simulink model "ec_datadict_buses"  (Simulink 10.0)
settings: Solver=FixedStepDiscrete  StartTime=0.0  StopTime=10  RelTol=1e-3  EnableMultiTasking=on
PreLoadFcn:
  | ec_data_fixpt_sc;
StartFcn:
  | tic
StopFcn:
  | toc
undefined symbols (not defined in the file): dfilt, ec_length, ec_window_len, Fs, magnitude, pic_frame_size, spkr_to_mic_filter, spkr_to_mic_gain
libraries: dspsrcs4 x24, simulink x14, dsparch4 x4, dspobslib x3, dspsnks4 x3, dspbuff3 x3, dspwin32 x2, dspsigops x2, dspmathops x2, dspadpt3 x1
settings Model: Creator=Kerry Schutz  LastModifiedBy=bhisma
settings DataIOCC: LimitDataPoints=on  SaveFormat=Structure  SignalLoggingSaveFormat=ModelDataLogs  SignalLogging=off
settings OptimizationCC: BlockReduction=off  DefaultParameterBehavior=Inlined  ExpressionDepthLimit=2147483647  InitFltsAndDblsToZero=on  LifeSpan=1  EfficientTunableParamExpr=on
settings DebuggingCC: SaveWithParameterizedLinksMsg=none  SolverPrmCheckMsg=warning  FcnCallInpInsideContextMsg=warning  StateNameClashWarn=warning
settings HardwareCC: ProdBitPerInt=16  ProdWordSize=16  ProdHWDeviceType=Specified
settings SFSimCC: SimUseLocalCustomCode=on  MATLABDynamicMemAlloc=off  CustomCodeUndefinedFunction=FilterOut
settings RTWCC: Description=Real-Time Workshop Embedded Coder (no auto configuration)  SystemTargetFile=ert.tlc  GenCodeOnly=on  TemplateMakefile=ert_default_tmf  GenerateReport=on  RTWUseLocalCustomCode=on  IncludeHyperlinkInReport=on  LaunchReport=on
settings CodeAppCC: IgnoreCustomStorageClasses=off  CustomSymbolStrType=$N$R$M  InternalIdentifier=Classic
settings ERTTargetCC: TargetFcnLib=ansi_tfl_tmw.mat  GenerateSampleERTMain=on  IncludeMdlTerminateFcn=off  SupportAbsoluteTime=off  SupportNonFinite=off  SupportComplex=off  InlinedParameterPlacement=NonHierarchical  ERTCustomFileTemplate=example_file_process.tlc  ConvertIfToSwitch=off  SuppressUnreachableDefaultCases=off

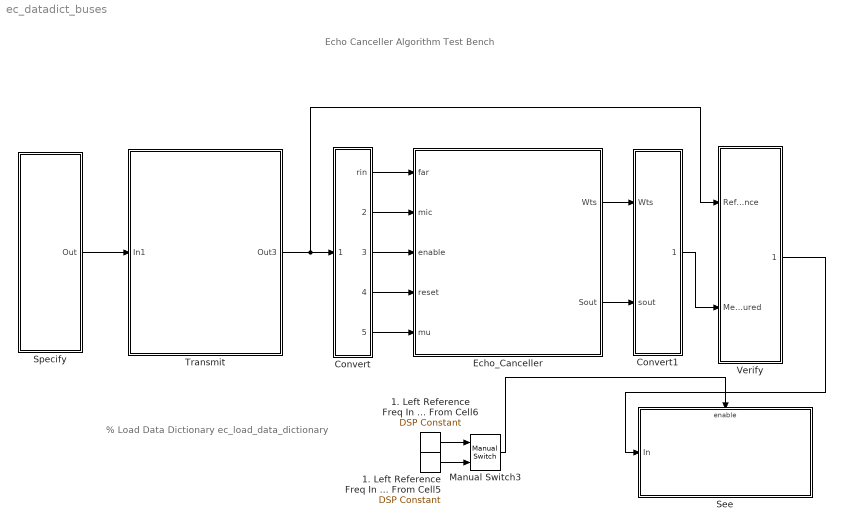
== system ec_datadict_buses ==
  note: Echo Canceller
      | Algorithm Test Bench
  note: % Load Data Dictionary
      | ec_load_data_dictionary
  1. Left Reference Freq In Hz From Cell5 : dspsrcs4/DSP Constant  SystemSampleTime=-1  Value=0  SampleMode=Discrete  discreteOutput=Sample-based  continuousOutput=Sample-based  sampTime=pic_frame_size/Fs  framePeriod=pic_frame_size/Fs  dataType=double  isSigned=on  wordLen=16  udDataType=sfix(16)  fracBitsMode=Best precision  numFracBits=15  InterpretAs1D=-inf  Ts=-inf  FramebasedOutput=-inf
      settings: SourceProductName=DSP System Toolbox  SourceProductBaseCode=DS  additionalParams=on
  1. Left Reference Freq In Hz From Cell6 : dspsrcs4/DSP Constant  SystemSampleTime=-1  Value=1  SampleMode=Discrete  discreteOutput=Sample-based  continuousOutput=Sample-based  sampTime=pic_frame_size/Fs  framePeriod=pic_frame_size/Fs  dataType=double  isSigned=on  wordLen=16  udDataType=sfix(16)  fracBitsMode=Best precision  numFracBits=15  InterpretAs1D=-inf  Ts=-inf  FramebasedOutput=-inf
      settings: SourceProductName=DSP System Toolbox  SourceProductBaseCode=DS  additionalParams=on
  Convert : Subsystem
  Convert1 : Subsystem
  Echo_Canceller : Subsystem  MinMaxOverflowLogging=MinMaxAndOverflow
      mask Display: image(imread('dsp_art.bmp'))
  Manual Switch3 : simulink/Signal Routing/Manual Switch  SystemSampleTime=-1  sw=1  action=0  varsize=off
      settings: SourceProductName=Simulink  SourceProductBaseCode=SL
  See : Subsystem
      mask Display: image(imread('visualizations.bmp'))
  Specify : Subsystem
      mask Display: image(imread('tests.bmp'))
  Transmit : Subsystem
      mask Display: image(imread('trans_path.bmp'))
  Verify : Subsystem
      mask Display: image(imread('verifications.bmp'))
  wires:
  Specify/1(Out) -> Transmit/1(In1)
  Transmit/1(Out3) -> Convert/1("  "), Verify/1(Reference)
  Convert/1(rin) -> Echo_Canceller/1(" far ")
  Convert/2(sin) -> Echo_Canceller/2("  mic")
  Convert/3(enable) -> Echo_Canceller/3(" enable")
  Echo_Canceller/1(Wts) -> Convert1/1(Wts)
  Echo_Canceller/2(Sout) -> Convert1/2(sout)
  Convert1/1(" ") -> Verify/2(Measured)
  Verify/1("  ") -> See/1(In)
  Convert/5(mu) -> Echo_Canceller/5(mu)
  Convert/4(reset) -> Echo_Canceller/4(reset)
  Manual Switch3/1 -> See/Enable
  1. Left Reference Freq In Hz From Cell5/1 -> Manual Switch3/2
  1. Left Reference Freq In Hz From Cell6/1 -> Manual Switch3/1

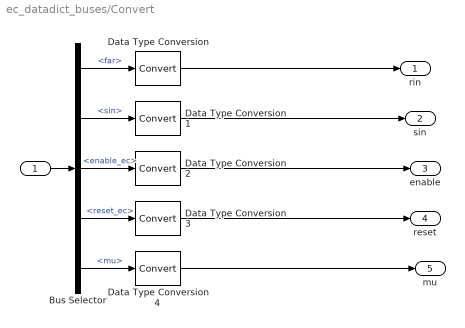
== system ec_datadict_buses/Convert ==
  "  " : Inport
  Bus Selector : BusSelector  OutputSignals=far,sin,enable_ec,reset_ec,mu
  Data Type Conversion{,1..4} (5 alike) : DataTypeConversion  SaturateOnIntegerOverflow=on
  rin : Outport
  sin : Outport  Port=2
  enable : Outport  Port=3
  reset : Outport  Port=4
  mu : Outport  Port=5
  wires:
  Bus Selector/1 -> Data Type Conversion/1  "<far>"
  Bus Selector/2 -> Data Type Conversion1/1  "<sin>"
  "  "/1 -> Bus Selector/1
  Data Type Conversion1/1 -> sin/1
  Data Type Conversion/1 -> rin/1
  Bus Selector/3 -> Data Type Conversion2/1  "<enable_ec>"
  Data Type Conversion2/1 -> enable/1
  Bus Selector/4 -> Data Type Conversion3/1  "<reset_ec>"
  Data Type Conversion3/1 -> reset/1
  Bus Selector/5 -> Data Type Conversion4/1  "<mu>"
  Data Type Conversion4/1 -> mu/1

== system ec_datadict_buses/Convert1 ==
  Wts : Inport
  sout : Inport  Port=2
  Bus Creator : BusCreator  Inputs=2
  Data Type Conversion : DataTypeConversion  OutDataTypeStr=double  SaturateOnIntegerOverflow=on
  Data Type Conversion1 : DataTypeConversion  OutDataTypeStr=double  SaturateOnIntegerOverflow=on
  " " : Outport
  wires:
  Wts/1 -> Data Type Conversion/1
  Bus Creator/1 -> " "/1
  sout/1 -> Data Type Conversion1/1
  Data Type Conversion/1 -> Bus Creator/1  "Wts"
  Data Type Conversion1/1 -> Bus Creator/2  "sout"

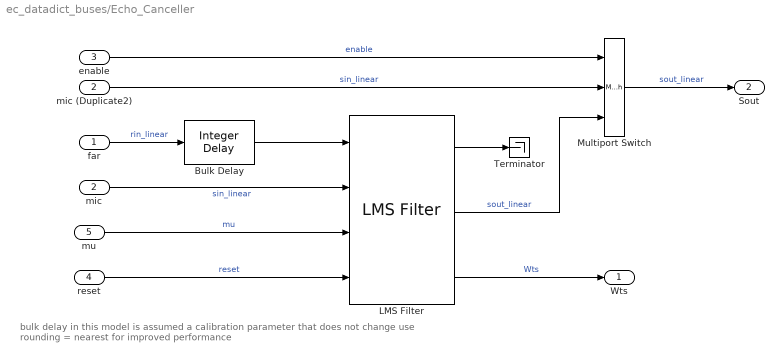
== system ec_datadict_buses/Echo_Canceller ==
  note: bulk delay in this model is assumed a calibration parameter that does not change
      | use rounding = nearest for improved performance
  " far " : Inport
  "  mic" : Inport  Port=2
  " enable" : Inport  Port=3
  reset : Inport  Port=4
  mu : Inport  Port=5
  "  mic (Duplicate2)" : InportShadow  Port=2
  Bulk Delay : dspobslib/Integer Delay  delay=spkr_to_mic_delay % this compensates for the delay in the filter and the spkr to mic path  ic=0  reset_popup=None
      settings: SourceProductName=DSP System Toolbox  SourceProductBaseCode=DS
  LMS Filter : dspadpt3/LMS Filter  Algo=LMS  L=ec_length  stepflag=Input port  mu=0.1  leakage=1.0  ic=0  Adapt=off  resetflag=Non-zero sample  weights=on  addnparflag=off  roundingMode=Nearest  overflowMode=off  secondCoeffMode=Binary point scaling  secondCoeffWordLength=2  secondCoeffFracLength=15  memoryMode=Binary point scaling  memoryWordLength=LMS_Wts_WordLen  memoryFracLength=LMS_Wts_FracLen  prodOutputMode=Binary point scaling  prodOutputWordLength=LMS_Prod_WordLen  prodOutputFracLength=20  prodOutput2Mode=Binary point scaling  prodOutput2FracLength=LMS_Prod_FracLen  prodOutput3Mode=Binary point scaling  prodOutput3FracLength=LMS_Prod_FracLen  prodOutput4Mode=Binary point scaling  prodOutput4FracLength=LMS_Prod_FracLen  quotientMode=Binary point scaling  quotientFracLength=20  accumMode=Binary point scaling  accumWordLength=LMS_Accum_WordLen  accumFracLength=20  accum2Mode=Binary point scaling  accum2FracLength=LMS_Accum_FracLen
      settings: SourceProductName=DSP System Toolbox  SourceProductBaseCode=DS
  Multiport Switch : MultiPortSwitch  DataPortOrder=Zero-based contiguous  Inputs=2  zeroidx=on
  Terminator : Terminator
  Wts : Outport
  Sout : Outport  Port=2
  wires:
  " far "/1 -> Bulk Delay/1  "rin_linear"
  "  mic"/1 -> LMS Filter/2  "sin_linear"
  LMS Filter/3 -> Wts/1  "Wts"
  LMS Filter/1 -> Terminator/1
  " enable"/1 -> Multiport Switch/1  "enable"
  LMS Filter/2 -> Multiport Switch/3  "sout_linear"
  "  mic (Duplicate2)"/1 -> Multiport Switch/2  "sin_linear"
  reset/1 -> LMS Filter/4  "reset"
  Multiport Switch/1 -> Sout/1  "sout_linear"
  mu/1 -> LMS Filter/3  "mu"
  Bulk Delay/1 -> LMS Filter/1

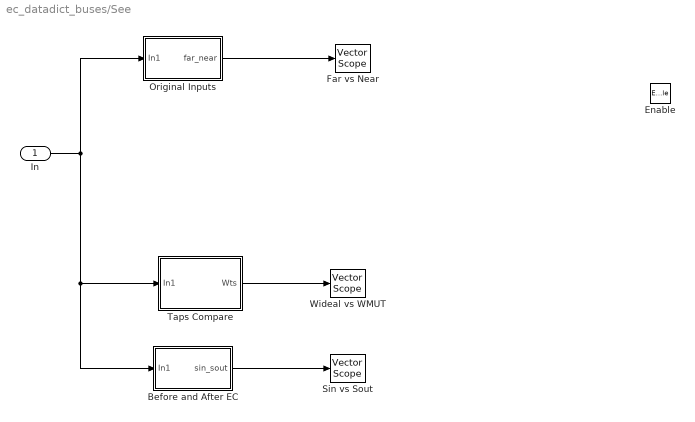
== system ec_datadict_buses/See ==
  In : Inport
  Enable : EnablePort
  Before and After EC : Subsystem
  Far vs Near : dspsnks4/Vector Scope  ScopeProperties=on  Domain=Time  HorizSpan=1  DisplayProperties=off  AxisGrid=on  Memory=off  FrameNumber=on  AxisLegend=off  AxisZoom=off  OpenScopeAtSimStart=on  OpenScopeImmediately=off  FigPos=[41 300 287 179]  AxisProperties=off  XUnits=Hertz  XRange=[0...Fs/2]  InheritXIncr=on  XIncr=1  XLabel=Time  XLimit=Auto  XMin=0  XMax=1  XStart=0  YUnits=dB  YLabel=Amplitude  LineProperties=off  LineColors=r|g
      settings: SourceProductName=DSP System Toolbox  SourceProductBaseCode=DS  YMin=-0.904474745892036  YMax=0.903014948842516
  Original Inputs : Subsystem
  Sin vs Sout : dspsnks4/Vector Scope  ScopeProperties=on  Domain=Time  HorizSpan=1  DisplayProperties=off  AxisGrid=on  Memory=off  FrameNumber=on  AxisLegend=off  AxisZoom=off  OpenScopeAtSimStart=on  OpenScopeImmediately=off  FigPos=[339 300 287 179]  AxisProperties=off  XUnits=Hertz  XRange=[0...Fs/2]  InheritXIncr=on  XIncr=1  XLabel=Time  XLimit=Auto  XMin=0  XMax=1  XStart=0  YUnits=dB  YLabel=Amplitude  LineProperties=off  LineColors=r|g
      settings: SourceProductName=DSP System Toolbox  SourceProductBaseCode=DS  YMin=-0.904474745892036  YMax=0.903014948842516
  Taps Compare : Subsystem
  Wideal vs WMUT : dspsnks4/Vector Scope  ScopeProperties=on  Domain=Time  HorizSpan=1  DisplayProperties=off  AxisGrid=on  Memory=off  FrameNumber=on  AxisLegend=off  AxisZoom=off  OpenScopeAtSimStart=on  OpenScopeImmediately=off  FigPos=[637 300 318 179]  AxisProperties=off  XUnits=Hertz  XRange=[0...Fs/2]  InheritXIncr=on  XIncr=1  XLabel=Time  XLimit=User-defined  XMin=4  XMax=6  XStart=0  YUnits=dB  YLabel=Amplitude  LineProperties=off  LineColors=r|g
      settings: SourceProductName=DSP System Toolbox  SourceProductBaseCode=DS  YMin=-0.0718456241378401  YMax=0.392086848285075
  wires:
  Original Inputs/1(far_near) -> Far vs Near/1
  In/1 -> Original Inputs/1(In1), Taps Compare/1(In1), Before and After EC/1(In1)
  Taps Compare/1(Wts) -> Wideal vs WMUT/1
  Before and After EC/1(sin_sout) -> Sin vs Sout/1

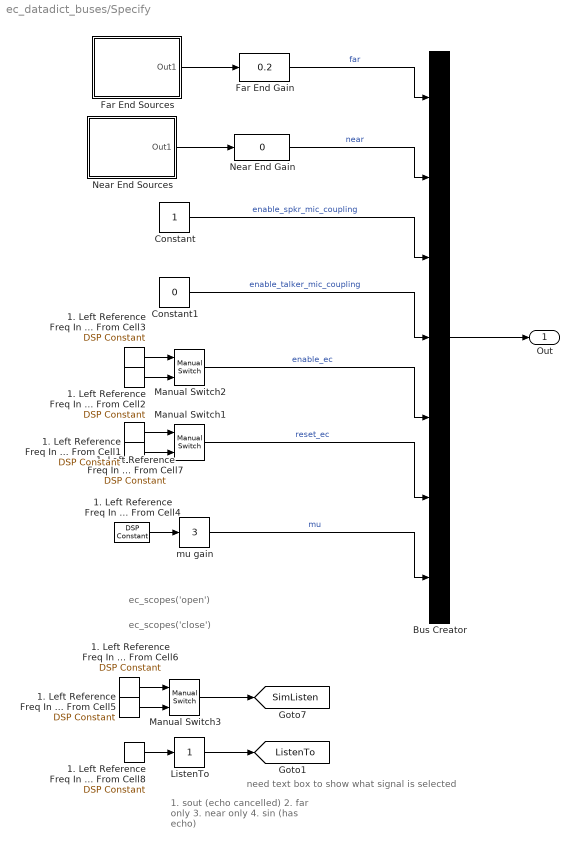
== system ec_datadict_buses/Specify ==
  note: ec_scopes('open')
  note: ec_scopes('close')
  note: need text box to show what signal is selected
  note: 1. sout (echo cancelled)
      | 2. far only
      | 3. near only
      | 4. sin (has echo)
  1. Left Reference Freq In Hz From Cell1 : dspsrcs4/DSP Constant  SystemSampleTime=-1  Value=0  SampleMode=Discrete  discreteOutput=Sample-based  continuousOutput=Sample-based  sampTime=pic_frame_size/Fs  framePeriod=pic_frame_size/Fs  dataType=double  isSigned=on  wordLen=16  udDataType=sfix(16)  fracBitsMode=Best precision  numFracBits=15  InterpretAs1D=-inf  Ts=-inf  FramebasedOutput=-inf
      settings: SourceProductName=DSP System Toolbox  SourceProductBaseCode=DS  additionalParams=on
  1. Left Reference Freq In Hz From Cell2 : dspsrcs4/DSP Constant  SystemSampleTime=-1  Value=0  SampleMode=Discrete  discreteOutput=Sample-based  continuousOutput=Sample-based  sampTime=pic_frame_size/Fs  framePeriod=pic_frame_size/Fs  dataType=double  isSigned=on  wordLen=16  udDataType=sfix(16)  fracBitsMode=Best precision  numFracBits=15  InterpretAs1D=-inf  Ts=-inf  FramebasedOutput=-inf
      settings: SourceProductName=DSP System Toolbox  SourceProductBaseCode=DS  additionalParams=on
  1. Left Reference Freq In Hz From Cell3 : dspsrcs4/DSP Constant  SystemSampleTime=-1  Value=1  SampleMode=Discrete  discreteOutput=Sample-based  continuousOutput=Sample-based  sampTime=pic_frame_size/Fs  framePeriod=pic_frame_size/Fs  dataType=double  isSigned=on  wordLen=16  udDataType=sfix(16)  fracBitsMode=Best precision  numFracBits=15  InterpretAs1D=-inf  Ts=-inf  FramebasedOutput=-inf
      settings: SourceProductName=DSP System Toolbox  SourceProductBaseCode=DS  additionalParams=on
  1. Left Reference Freq In Hz From Cell4 : dspsrcs4/DSP Constant  SystemSampleTime=-1  Value=.001  SampleMode=Discrete  discreteOutput=Sample-based  continuousOutput=Sample-based  sampTime=pic_frame_size/Fs  framePeriod=2  dataType=double  isSigned=on  wordLen=16  udDataType=sfix(16)  fracBitsMode=Best precision  numFracBits=15  InterpretAs1D=-inf  Ts=-inf  FramebasedOutput=-inf
      settings: SourceProductName=DSP System Toolbox  SourceProductBaseCode=DS  additionalParams=on
  1. Left Reference Freq In Hz From Cell5 : dspsrcs4/DSP Constant  SystemSampleTime=-1  Value=0  SampleMode=Discrete  discreteOutput=Sample-based  continuousOutput=Sample-based  sampTime=pic_frame_size/Fs  framePeriod=pic_frame_size/Fs  dataType=double  isSigned=on  wordLen=16  udDataType=sfix(16)  fracBitsMode=Best precision  numFracBits=15  InterpretAs1D=-inf  Ts=-inf  FramebasedOutput=-inf
      settings: SourceProductName=DSP System Toolbox  SourceProductBaseCode=DS  additionalParams=on
  1. Left Reference Freq In Hz From Cell6 : dspsrcs4/DSP Constant  SystemSampleTime=-1  Value=1  SampleMode=Discrete  discreteOutput=Sample-based  continuousOutput=Sample-based  sampTime=pic_frame_size/Fs  framePeriod=pic_frame_size/Fs  dataType=double  isSigned=on  wordLen=16  udDataType=sfix(16)  fracBitsMode=Best precision  numFracBits=15  InterpretAs1D=-inf  Ts=-inf  FramebasedOutput=-inf
      settings: SourceProductName=DSP System Toolbox  SourceProductBaseCode=DS  additionalParams=on
  1. Left Reference Freq In Hz From Cell7 : dspsrcs4/DSP Constant  SystemSampleTime=-1  Value=1  SampleMode=Discrete  discreteOutput=Sample-based  continuousOutput=Sample-based  sampTime=pic_frame_size/Fs  framePeriod=pic_frame_size/Fs  dataType=double  isSigned=on  wordLen=16  udDataType=sfix(16)  fracBitsMode=Best precision  numFracBits=15  InterpretAs1D=-inf  Ts=-inf  FramebasedOutput=-inf
      settings: SourceProductName=DSP System Toolbox  SourceProductBaseCode=DS  additionalParams=on
  1. Left Reference Freq In Hz From Cell8 : dspsrcs4/DSP Constant  SystemSampleTime=-1  Value=1  SampleMode=Discrete  discreteOutput=Sample-based  continuousOutput=Sample-based  sampTime=pic_frame_size/Fs  framePeriod=2  dataType=double  isSigned=on  wordLen=16  udDataType=sfix(16)  fracBitsMode=Best precision  numFracBits=15  InterpretAs1D=-inf  Ts=-inf  FramebasedOutput=-inf
      settings: SourceProductName=DSP System Toolbox  SourceProductBaseCode=DS  additionalParams=on
  Bus Creator : BusCreator  Inputs=7
  Constant : Constant
  Constant1 : Constant  Value=0
  Far End Gain : simulink/Math Operations/Slider Gain  SystemSampleTime=-1  low=0  gain=0.2  high=10
  Far End Sources : Subsystem
  ListenTo : simulink/Math Operations/Slider Gain  SystemSampleTime=-1  low=0  gain=1  high=10
  Manual Switch1 : simulink/Signal Routing/Manual Switch  SystemSampleTime=-1  sw=0  action=0  varsize=off
      settings: SourceProductName=Simulink  SourceProductBaseCode=SL
  Manual Switch2 : simulink/Signal Routing/Manual Switch  SystemSampleTime=-1  sw=1  action=0  varsize=off
      settings: SourceProductName=Simulink  SourceProductBaseCode=SL
  Manual Switch3 : simulink/Signal Routing/Manual Switch  SystemSampleTime=-1  sw=0  action=0  varsize=off
      settings: SourceProductName=Simulink  SourceProductBaseCode=SL
  Near End Gain : simulink/Math Operations/Slider Gain  SystemSampleTime=-1  low=0  gain=0  high=10
  Near End Sources : Subsystem
  mu gain : simulink/Math Operations/Slider Gain  SystemSampleTime=-1  low=0  gain=3  high=100
  Out : Outport
  tag scope: ListenTo=global, SimListen=global
  wires:
  Far End Sources/1(Out1) -> Far End Gain/1
  Near End Sources/1(Out1) -> Near End Gain/1
  Far End Gain/1 -> Bus Creator/1  "far"
  Near End Gain/1 -> Bus Creator/2  "near"
  Bus Creator/1 -> Out/1
  Constant/1 -> Bus Creator/3  "enable_spkr_mic_coupling"
  Constant1/1 -> Bus Creator/4  "enable_talker_mic_coupling"
  1. Left Reference Freq In Hz From Cell1/1 -> Manual Switch1/2
  1. Left Reference Freq In Hz From Cell7/1 -> Manual Switch1/1
  Manual Switch1/1 -> Bus Creator/6  "reset_ec"
  1. Left Reference Freq In Hz From Cell2/1 -> Manual Switch2/2
  1. Left Reference Freq In Hz From Cell3/1 -> Manual Switch2/1
  Manual Switch2/1 -> Bus Creator/5  "enable_ec"
  1. Left Reference Freq In Hz From Cell4/1 -> mu gain/1
  mu gain/1 -> Bus Creator/7  "mu"
  1. Left Reference Freq In Hz From Cell5/1 -> Manual Switch3/2
  1. Left Reference Freq In Hz From Cell6/1 -> Manual Switch3/1
  Manual Switch3/1 -> [SimListen]
  ListenTo/1 -> [ListenTo]
  1. Left Reference Freq In Hz From Cell8/1 -> ListenTo/1

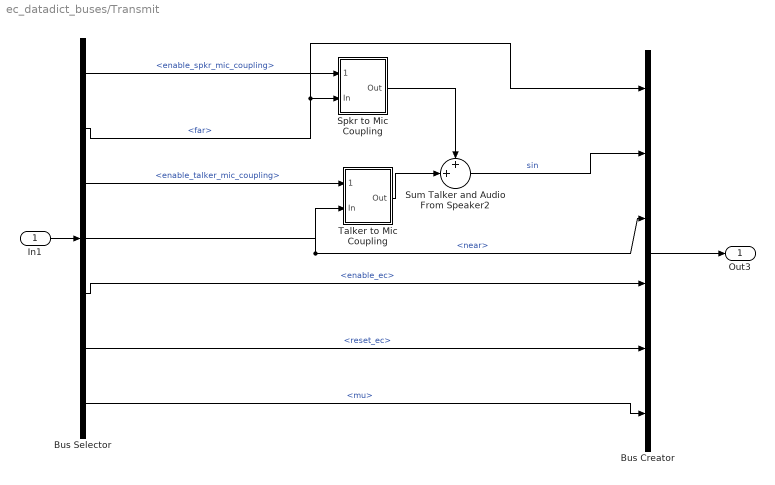
== system ec_datadict_buses/Transmit ==
  In1 : Inport
  Bus Creator : BusCreator  Inputs=6
  Bus Selector : BusSelector  OutputSignals=enable_spkr_mic_coupling,far,enable_talker_mic_coupling,near,enable_ec,reset_ec,mu
  Spkr to Mic Coupling : Subsystem
  Sum Talker and Audio From Speaker2 : Sum  Inputs=++|  SaturateOnIntegerOverflow=on  OutDataTypeStr=Inherit: Same as first input
  Talker to Mic Coupling : Subsystem
  Out3 : Outport
  wires:
  In1/1 -> Bus Selector/1
  Bus Creator/1 -> Out3/1
  Bus Selector/2 -> Spkr to Mic Coupling/2(In), Bus Creator/1  "<far>"
  Bus Selector/1 -> Spkr to Mic Coupling/1(enable)  "<enable_spkr_mic_coupling>"
  Bus Selector/3 -> Talker to Mic Coupling/1(enable)  "<enable_talker_mic_coupling>"
  Bus Selector/4 -> Talker to Mic Coupling/2(In), Bus Creator/3  "<near>"
  Spkr to Mic Coupling/1(Out) -> Sum Talker and Audio From Speaker2/1
  Talker to Mic Coupling/1(Out) -> Sum Talker and Audio From Speaker2/2
  Bus Selector/5 -> Bus Creator/4  "<enable_ec>"
  Bus Selector/6 -> Bus Creator/5  "<reset_ec>"
  Bus Selector/7 -> Bus Creator/6  "<mu>"
  Sum Talker and Audio From Speaker2/1 -> Bus Creator/2  "sin"

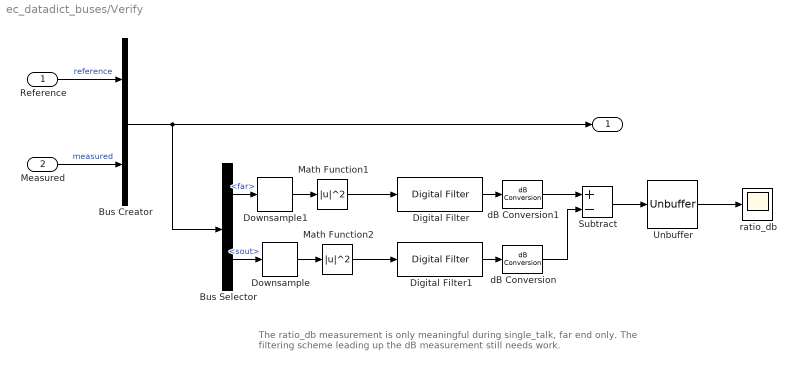
== system ec_datadict_buses/Verify ==
  note: The ratio_db measurement is only meaningful during single_talk, far end only.
      | The filtering scheme leading up the dB measurement still needs work.
  Reference : Inport
  Measured : Inport  Port=2
  Bus Creator : BusCreator  Inputs=2
  Bus Selector : BusSelector  OutputSignals=reference.far,measured.sout
  Digital Filter : dsparch4/Digital Filter  TypePopup=FIR (all zeros)  IIRFiltStruct=Direct form II transposed  AllPoleFiltStruct=Direct form  FIRFiltStruct=Direct form  CoeffSource=Specify via dialog  NumCoeffs=[ones(1,80)/80]  DenCoeffs=[1 0.1]  BiQuadCoeffs=[1 0.3 0.4 1 0.1 0.2]  LatticeCoeffs=[0.2 0.4]  denIgnore=on  FiltPerSampPopup=One filter per frame  IC=0  ICnum=0  ICden=0  roundingMode=Floor  overflowMode=off  ScaleValues=1  scaleValueFracLength=14  stageInFracLength=15  stageOutFracLength=15  FilterSource=Specify via dialog  dfiltObjectName=dfilt.dffir([1 2 1])
      settings: SourceProductName=DSP System Toolbox  SourceProductBaseCode=DS
  Digital Filter1 : dsparch4/Digital Filter  TypePopup=FIR (all zeros)  IIRFiltStruct=Direct form II transposed  AllPoleFiltStruct=Direct form  FIRFiltStruct=Direct form  CoeffSource=Specify via dialog  NumCoeffs=[ones(1,80)/80]  DenCoeffs=[1 0.1]  BiQuadCoeffs=[1 0.3 0.4 1 0.1 0.2]  LatticeCoeffs=[0.2 0.4]  denIgnore=on  FiltPerSampPopup=One filter per frame  IC=0  ICnum=0  ICden=0  roundingMode=Floor  overflowMode=off  ScaleValues=1  scaleValueFracLength=14  stageInFracLength=15  stageOutFracLength=15  FilterSource=Specify via dialog  dfiltObjectName=dfilt.dffir([1 2 1])
      settings: SourceProductName=DSP System Toolbox  SourceProductBaseCode=DS
  Downsample : dspsigops/Downsample  N=10  phase=0  ic=0  smode=Allow multirate  fmode=Maintain input frame size
      settings: SourceProductName=DSP System Toolbox  SourceProductBaseCode=DS
  Downsample1 : dspsigops/Downsample  N=10  phase=0  ic=0  smode=Allow multirate  fmode=Maintain input frame size
      settings: SourceProductName=DSP System Toolbox  SourceProductBaseCode=DS
  Math Function1 : Math  Operator=magnitude^2  SaturateOnIntegerOverflow=on
  Math Function2 : Math  Operator=magnitude^2  SaturateOnIntegerOverflow=on
  Subtract : Sum  Inputs=+-
  Unbuffer : dspbuff3/Unbuffer  ic=0
      settings: SourceProductName=DSP System Toolbox  SourceProductBaseCode=DS
  dB Conversion : dspmathops/dB Conversion  SystemSampleTime=-1  dBtype=dB  intype=Power  R=1  fuzz=on
      settings: SourceProductName=DSP System Toolbox
  dB Conversion1 : dspmathops/dB Conversion  SystemSampleTime=-1  dBtype=dB  intype=Power  R=1  fuzz=on
      settings: SourceProductName=DSP System Toolbox
  ratio_db : Scope
  "  " : Outport
  wires:
  Reference/1 -> Bus Creator/1  "reference"
  Measured/1 -> Bus Creator/2  "measured"
  Bus Creator/1 -> "  "/1, Bus Selector/1
  Bus Selector/1 -> Downsample1/1  "<far>"
  Bus Selector/2 -> Downsample/1  "<sout>"
  Unbuffer/1 -> ratio_db/1
  Math Function1/1 -> Digital Filter/1
  Digital Filter/1 -> dB Conversion1/1
  Math Function2/1 -> Digital Filter1/1
  Digital Filter1/1 -> dB Conversion/1
  Subtract/1 -> Unbuffer/1
  Downsample/1 -> Math Function2/1
  Downsample1/1 -> Math Function1/1
  dB Conversion/1 -> Subtract/2
  dB Conversion1/1 -> Subtract/1

== system ec_datadict_buses/See/Before and After EC ==
  In1 : Inport
  Bus Selector : BusSelector  OutputSignals=reference.sin,measured.sout
  Matrix Concatenate1 : Concatenate  Mode=Multidimensional array  ConcatenateDimension=2
  sin_sout : Outport
  wires:
  Matrix Concatenate1/1 -> sin_sout/1
  In1/1 -> Bus Selector/1
  Bus Selector/2 -> Matrix Concatenate1/2  "<sout>"
  Bus Selector/1 -> Matrix Concatenate1/1  "<sin>"

== system ec_datadict_buses/See/Original Inputs ==
  In1 : Inport
  Bus Selector : BusSelector  OutputSignals=reference.far,reference.near
  Matrix Concatenate1 : Concatenate  Mode=Multidimensional array  ConcatenateDimension=2
  far_near : Outport
  wires:
  Bus Selector/1 -> Matrix Concatenate1/1  "<far>"
  Bus Selector/2 -> Matrix Concatenate1/2  "<near>"
  In1/1 -> Bus Selector/1
  Matrix Concatenate1/1 -> far_near/1

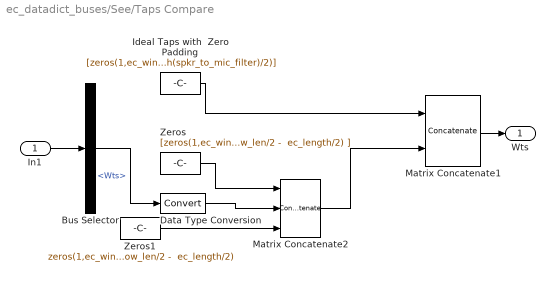
== system ec_datadict_buses/See/Taps Compare ==
  In1 : Inport
  Bus Selector : BusSelector  OutputSignals=measured.Wts
  Data Type Conversion : DataTypeConversion
  Ideal Taps with  Zero Padding : Constant  Value="[zeros(1,ec_window_len/2 -  length(spkr_to_mic_filter)/2) spkr_to_mic_filter zeros(1,ec_window_len/2 -  length(spkr_to_mic_filter)/2)]"  SampleTime=pic_frame_size/Fs  FramePeriod=pic_frame_size/Fs
      settings: SamplingMode=Frame based
  Matrix Concatenate1 : Concatenate  Mode=Multidimensional array  ConcatenateDimension=2
  Matrix Concatenate2 : Concatenate  NumInputs=3
  Zeros : Constant  Value="[zeros(1,ec_window_len/2 -  ec_length/2) ]"  SampleTime=pic_frame_size/Fs  FramePeriod=pic_frame_size/Fs
      settings: SamplingMode=Frame based
  Zeros1 : Constant  Value="zeros(1,ec_window_len/2 -  ec_length/2)"  SampleTime=pic_frame_size/Fs  FramePeriod=pic_frame_size/Fs
      settings: SamplingMode=Frame based
  Wts : Outport
  wires:
  Ideal Taps with  Zero Padding/1 -> Matrix Concatenate1/1
  In1/1 -> Bus Selector/1
  Matrix Concatenate1/1 -> Wts/1
  Bus Selector/1 -> Data Type Conversion/1  "<Wts>"
  Zeros/1 -> Matrix Concatenate2/1
  Zeros1/1 -> Matrix Concatenate2/3
  Matrix Concatenate2/1 -> Matrix Concatenate1/2
  Data Type Conversion/1 -> Matrix Concatenate2/2

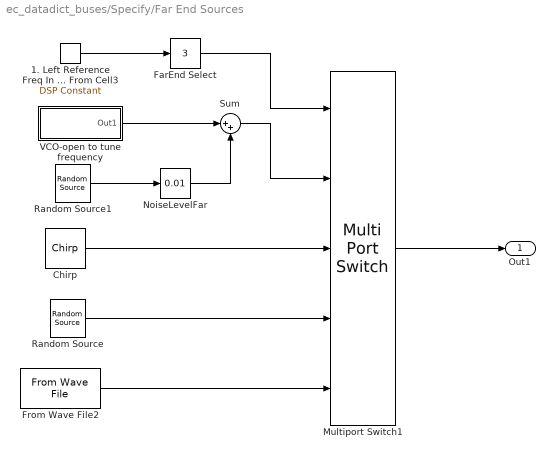
== system ec_datadict_buses/Specify/Far End Sources ==
  1. Left Reference Freq In Hz From Cell3 : dspsrcs4/DSP Constant  SystemSampleTime=-1  Value=1  SampleMode=Discrete  discreteOutput=Sample-based  continuousOutput=Sample-based  sampTime=pic_frame_size/Fs  framePeriod=2  dataType=double  isSigned=on  wordLen=16  udDataType=sfix(16)  fracBitsMode=Best precision  numFracBits=15  InterpretAs1D=-inf  Ts=-inf  FramebasedOutput=-inf
      settings: SourceProductName=DSP System Toolbox  SourceProductBaseCode=DS  additionalParams=on
  Chirp : dspsrcs4/Chirp  sweep=Linear  mode=Unidirectional  f0=100  f1=4000  t1=pic_frame_size/Fs  Tsweep=pic_frame_size/Fs  phase=0  Ts=1/Fs  spf=pic_frame_size  datatype=Double
      settings: SourceProductName=DSP System Toolbox
  FarEnd Select : simulink/Math Operations/Slider Gain  SystemSampleTime=-1  low=0  gain=3  high=10
  From Wave File2 : dspwin32/From Wave File  FileName=far_end.wav  SamplesPerFrame=80  MinBufSize=80  dType=double  bLoop=on  timesToPlay=inf  restartMode=immediately after last sample  firstSampleOutput=off  lastSampleOutput=off
      settings: SourceProductName=DSP System Toolbox  SourceProductBaseCode=DS
  Multiport Switch1 : MultiPortSwitch  Inputs=4  SampleTime=pic_frame_size/Fs
  NoiseLevelFar : simulink/Math Operations/Slider Gain  SystemSampleTime=-1  low=0  gain=0.01  high=1
  Random Source : dspsrcs4/Random Source  SrcType=Gaussian  NormMethod=Ziggurat  CltLength=12  MinVal=0  MaxVal=1  MeanVal=0  VarVal=1  RepMode=Not repeatable  rawSeed=1  IsInherit=off  SampMode=Discrete  SampTime=1/Fs  SampFrame=pic_frame_size  DataType=Double  OutComplex=Real
  Random Source1 : dspsrcs4/Random Source  SrcType=Gaussian  NormMethod=Ziggurat  CltLength=12  MinVal=0  MaxVal=1  MeanVal=0  VarVal=1  RepMode=Not repeatable  rawSeed=1  IsInherit=off  SampMode=Discrete  SampTime=1/Fs  SampFrame=pic_frame_size  DataType=Double  OutComplex=Real
  Sum : Sum  Inputs=|++
  VCO-open to tune frequency : Subsystem
  Out1 : Outport
  wires:
  VCO-open to tune frequency/1(Out1) -> Sum/1
  Multiport Switch1/1 -> Out1/1
  From Wave File2/1 -> Multiport Switch1/5
  Chirp/1 -> Multiport Switch1/3
  Random Source/1 -> Multiport Switch1/4
  1. Left Reference Freq In Hz From Cell3/1 -> FarEnd Select/1
  FarEnd Select/1 -> Multiport Switch1/1
  Sum/1 -> Multiport Switch1/2
  Random Source1/1 -> NoiseLevelFar/1
  NoiseLevelFar/1 -> Sum/2

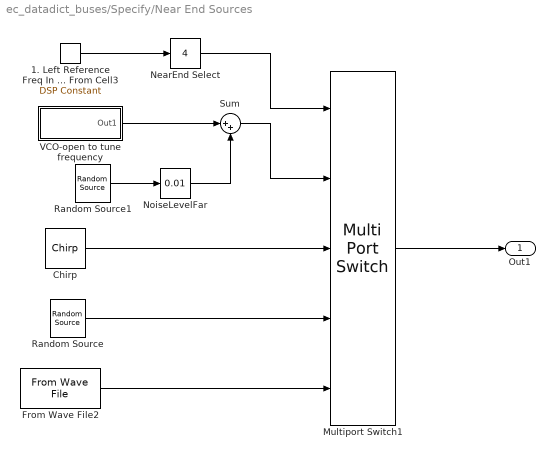
== system ec_datadict_buses/Specify/Near End Sources ==
  1. Left Reference Freq In Hz From Cell3 : dspsrcs4/DSP Constant  SystemSampleTime=-1  Value=1  SampleMode=Discrete  discreteOutput=Sample-based  continuousOutput=Sample-based  sampTime=pic_frame_size/Fs  framePeriod=2  dataType=double  isSigned=on  wordLen=16  udDataType=sfix(16)  fracBitsMode=Best precision  numFracBits=15  InterpretAs1D=-inf  Ts=-inf  FramebasedOutput=-inf
      settings: SourceProductName=DSP System Toolbox  SourceProductBaseCode=DS  additionalParams=on
  Chirp : dspsrcs4/Chirp  sweep=Linear  mode=Unidirectional  f0=100  f1=4000  t1=pic_frame_size/Fs  Tsweep=pic_frame_size/Fs  phase=0  Ts=1/Fs  spf=pic_frame_size  datatype=Double
      settings: SourceProductName=DSP System Toolbox
  From Wave File2 : dspwin32/From Wave File  FileName=near_end.wav  SamplesPerFrame=80  MinBufSize=80  dType=double  bLoop=on  timesToPlay=inf  restartMode=immediately after last sample  firstSampleOutput=off  lastSampleOutput=off
      settings: SourceProductName=DSP System Toolbox  SourceProductBaseCode=DS
  Multiport Switch1 : MultiPortSwitch  Inputs=4  SampleTime=pic_frame_size/Fs
  NearEnd Select : simulink/Math Operations/Slider Gain  SystemSampleTime=-1  low=0  gain=4  high=10
  NoiseLevelFar : simulink/Math Operations/Slider Gain  SystemSampleTime=-1  low=0  gain=0.01  high=1
  Random Source : dspsrcs4/Random Source  SrcType=Gaussian  NormMethod=Ziggurat  CltLength=12  MinVal=0  MaxVal=1  MeanVal=0  VarVal=1  RepMode=Not repeatable  rawSeed=1  IsInherit=off  SampMode=Discrete  SampTime=1/Fs  SampFrame=pic_frame_size  DataType=Double  OutComplex=Real
  Random Source1 : dspsrcs4/Random Source  SrcType=Gaussian  NormMethod=Ziggurat  CltLength=12  MinVal=0  MaxVal=1  MeanVal=0  VarVal=1  RepMode=Not repeatable  rawSeed=1  IsInherit=off  SampMode=Discrete  SampTime=1/Fs  SampFrame=pic_frame_size  DataType=Double  OutComplex=Real
  Sum : Sum  Inputs=|++
  VCO-open to tune frequency : Subsystem
  Out1 : Outport
  wires:
  VCO-open to tune frequency/1(Out1) -> Sum/1
  Multiport Switch1/1 -> Out1/1
  From Wave File2/1 -> Multiport Switch1/5
  Chirp/1 -> Multiport Switch1/3
  Random Source/1 -> Multiport Switch1/4
  1. Left Reference Freq In Hz From Cell3/1 -> NearEnd Select/1
  NearEnd Select/1 -> Multiport Switch1/1
  Sum/1 -> Multiport Switch1/2
  Random Source1/1 -> NoiseLevelFar/1
  NoiseLevelFar/1 -> Sum/2

== system ec_datadict_buses/Transmit/Spkr to Mic Coupling ==
  enable : Inport
  In : Inport  Port=2
  Digital Filter Design : dsparch4/Digital Filter Design  SystemSampleTime=-1  mwdsp_browser_bugfix_var=off
  Gain : Gain  Gain=spkr_to_mic_gain
  Multiport Switch : MultiPortSwitch  DataPortOrder=Zero-based contiguous  Inputs=2  zeroidx=on
  Time Delay : dspobslib/Integer Delay  delay=spkr_to_mic_delay  ic=0  reset_popup=None
      settings: AttributesFormatString=-----------------------------------------------\ndelay = %<delay>\n-----------------------------------------------  SourceProductName=DSP System Toolbox  SourceProductBaseCode=DS
  Out : Outport
  wires:
  Digital Filter Design/1 -> Gain/1
  Time Delay/1 -> Digital Filter Design/1
  In/1 -> Time Delay/1, Multiport Switch/2
  Gain/1 -> Multiport Switch/3
  enable/1 -> Multiport Switch/1
  Multiport Switch/1 -> Out/1

== system ec_datadict_buses/Transmit/Talker to Mic Coupling ==
  enable : Inport
  In : Inport  Port=2
  Digital Filter Design : dsparch4/Digital Filter Design  SystemSampleTime=-1  mwdsp_browser_bugfix_var=off
  Gain : Gain  Gain=spkr_to_mic_gain
  Multiport Switch : MultiPortSwitch  DataPortOrder=Zero-based contiguous  Inputs=2  zeroidx=on
  Time Delay : dspobslib/Integer Delay  delay=talker_to_mic_delay  ic=0  reset_popup=None
      settings: AttributesFormatString=-----------------------------------------------\ndelay = %<delay>\n-----------------------------------------------  SourceProductName=DSP System Toolbox  SourceProductBaseCode=DS
  Out : Outport
  wires:
  Multiport Switch/1 -> Out/1
  enable/1 -> Multiport Switch/1
  Gain/1 -> Multiport Switch/3
  In/1 -> Time Delay/1, Multiport Switch/2
  Time Delay/1 -> Digital Filter Design/1
  Digital Filter Design/1 -> Gain/1

== system ec_datadict_buses/Specify/Far End Sources/VCO-open to tune frequency ==
  1. Left Reference Freq In Hz From Cell : dspsrcs4/DSP Constant  SystemSampleTime=-1  Value=1000  SampleMode=Discrete  discreteOutput=Sample-based  continuousOutput=Sample-based  sampTime=1/Fs  framePeriod=2  dataType=double  isSigned=on  wordLen=16  udDataType=sfix(16)  fracBitsMode=Best precision  numFracBits=15  InterpretAs1D=-inf  Ts=-inf  FramebasedOutput=-inf
      settings: SourceProductName=DSP System Toolbox  SourceProductBaseCode=DS  additionalParams=on
  Buffer2 : dspbuff3/Buffer  N=pic_frame_size  V=0  ic=0
      settings: SourceProductName=DSP System Toolbox  SourceProductBaseCode=DS
  Discrete-Time VCO : Subsystem  mask(Discrete-Time VCO){Ac=1, Fc=0, Kc=1, Ph=pi/2, ts=1/Fs}
      mask prompts: Ac "Output amplitude:"; Fc "Oscillation frequency (Hz):"; Kc "Input sensitivity:"; Ph "Initial phase (rad):"; ts "Sample time:"
      mask help: Generate a discrete-time output signal whose frequency changes in response to the amplitude variations of the input signal. The input signal must be a scalar.
      mask init:
      | if ((length(Ac)~=1) | (length(Fc)~=1) | (length(Kc)~=1) | (length(Ph)~=1) | (length(ts)~=1) |(length(Ph)~=1))error('Mask parameters must be scalar values.');end;
      | pi2=2*pi;
      mask Help: helpview(commbhelp)
      mask Display: disp('Discrete-Time\nVCO (rab)')
  FE FreqAdjust : simulink/Math Operations/Slider Gain  SystemSampleTime=-1  low=0  gain=1.1  high=5
  Out1 : Outport
  wires:
  Buffer2/1 -> Out1/1
  Discrete-Time VCO/1(out_1) -> Buffer2/1
  FE FreqAdjust/1 -> Discrete-Time VCO/1(in_1)
  1. Left Reference Freq In Hz From Cell/1 -> FE FreqAdjust/1

== system ec_datadict_buses/Specify/Near End Sources/VCO-open to tune frequency ==
  1. Left Reference Freq In Hz From Cell : dspsrcs4/DSP Constant  SystemSampleTime=-1  Value=1000  SampleMode=Discrete  discreteOutput=Sample-based  continuousOutput=Sample-based  sampTime=1/Fs  framePeriod=2  dataType=double  isSigned=on  wordLen=16  udDataType=sfix(16)  fracBitsMode=Best precision  numFracBits=15  InterpretAs1D=-inf  Ts=-inf  FramebasedOutput=-inf
      settings: SourceProductName=DSP System Toolbox  SourceProductBaseCode=DS  additionalParams=on
  Buffer2 : dspbuff3/Buffer  N=pic_frame_size  V=0  ic=0
      settings: SourceProductName=DSP System Toolbox  SourceProductBaseCode=DS
  Discrete-Time VCO : Subsystem  mask(Discrete-Time VCO){Ac=1, Fc=0, Kc=1, Ph=pi/2, ts=1/Fs}
      mask prompts: Ac "Output amplitude:"; Fc "Oscillation frequency (Hz):"; Kc "Input sensitivity:"; Ph "Initial phase (rad):"; ts "Sample time:"
      mask help: Generate a discrete-time output signal whose frequency changes in response to the amplitude variations of the input signal. The input signal must be a scalar.
      mask init:
      | if ((length(Ac)~=1) | (length(Fc)~=1) | (length(Kc)~=1) | (length(Ph)~=1) | (length(ts)~=1) |(length(Ph)~=1))error('Mask parameters must be scalar values.');end;
      | pi2=2*pi;
      mask Help: helpview(commbhelp)
      mask Display: disp('Discrete-Time\nVCO (rab)')
  NE FreqAdjust : simulink/Math Operations/Slider Gain  SystemSampleTime=-1  low=0  gain=0.5  high=5
  Out1 : Outport
  wires:
  Buffer2/1 -> Out1/1
  Discrete-Time VCO/1(out_1) -> Buffer2/1
  NE FreqAdjust/1 -> Discrete-Time VCO/1(in_1)
  1. Left Reference Freq In Hz From Cell/1 -> NE FreqAdjust/1

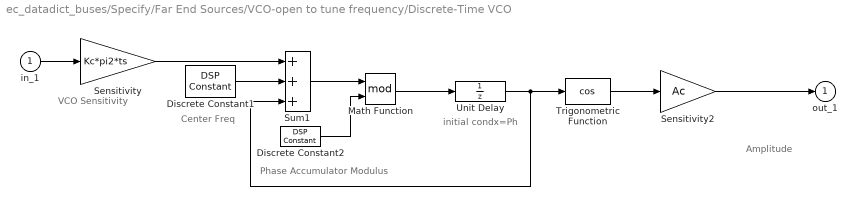
== system ec_datadict_buses/Specify/Far End Sources/VCO-open to tune frequency/Discrete-Time VCO ==
  note: Amplitude
  note: Phase Accumulator
      | Modulus
  note: Center Freq
  note: VCO Sensitivity
  note: initial condx=Ph
  in_1 : Inport
  Discrete Constant1 : dspsrcs4/DSP Constant  SystemSampleTime=-1  Value=Fc*pi2*ts  SampleMode=Discrete  discreteOutput=Sample-based (interpret vectors as 1-D)  continuousOutput=Sample-based  sampTime=1/8000  framePeriod=1/8000  dataType=Inherit via back propagation  isSigned=on  wordLen=16  udDataType=sfix(16)  fracBitsMode=Best precision  numFracBits=15  InterpretAs1D=on  Ts=1/8000  FramebasedOutput=off
      settings: SourceProductName=DSP System Toolbox  SourceProductBaseCode=DS  additionalParams=on
  Discrete Constant2 : dspsrcs4/DSP Constant  SystemSampleTime=-1  Value=pi2  SampleMode=Discrete  discreteOutput=Sample-based (interpret vectors as 1-D)  continuousOutput=Sample-based  sampTime=1/8000  framePeriod=1/8000  dataType=Inherit via back propagation  isSigned=on  wordLen=16  udDataType=sfix(16)  fracBitsMode=Best precision  numFracBits=15  InterpretAs1D=on  Ts=1/8000  FramebasedOutput=off
      settings: SourceProductName=DSP System Toolbox  SourceProductBaseCode=DS  additionalParams=on
  Math Function : Math  Operator=mod  SaturateOnIntegerOverflow=on
  Sensitivity : Gain  Gain=Kc*pi2*ts  SaturateOnIntegerOverflow=on  OutDataTypeStr=Inherit: Same as input  ParamDataTypeStr=Inherit: Same as input
  Sensitivity2 : Gain  Gain=Ac  SaturateOnIntegerOverflow=on  OutDataTypeStr=Inherit: Same as input  ParamDataTypeStr=Inherit: Same as input
  Sum1 : Sum  Inputs=+++  SaturateOnIntegerOverflow=on  InputSameDT=on  OutDataTypeStr=Inherit: Same as first input
  Trigonometric Function : Trigonometry  Operator=cos
  Unit Delay : UnitDelay  InitialCondition=Ph  SampleTime=ts
  out_1 : Outport  InitialOutput=0
  wires:
  Discrete Constant1/1 -> Sum1/2
  Sensitivity2/1 -> out_1/1
  Trigonometric Function/1 -> Sensitivity2/1
  Unit Delay/1 -> Trigonometric Function/1, Sum1/3
  Sensitivity/1 -> Sum1/1
  in_1/1 -> Sensitivity/1
  Math Function/1 -> Unit Delay/1
  Sum1/1 -> Math Function/1
  Discrete Constant2/1 -> Math Function/2

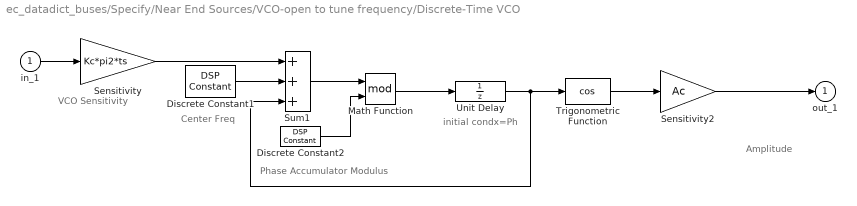
== system ec_datadict_buses/Specify/Near End Sources/VCO-open to tune frequency/Discrete-Time VCO ==
  note: Amplitude
  note: Phase Accumulator
      | Modulus
  note: Center Freq
  note: VCO Sensitivity
  note: initial condx=Ph
  in_1 : Inport
  Discrete Constant1 : dspsrcs4/DSP Constant  SystemSampleTime=-1  Value=Fc*pi2*ts  SampleMode=Discrete  discreteOutput=Sample-based (interpret vectors as 1-D)  continuousOutput=Sample-based  sampTime=1/8000  framePeriod=1/8000  dataType=Inherit via back propagation  isSigned=on  wordLen=16  udDataType=sfix(16)  fracBitsMode=Best precision  numFracBits=15  InterpretAs1D=on  Ts=1/8000  FramebasedOutput=off
      settings: SourceProductName=DSP System Toolbox  SourceProductBaseCode=DS  additionalParams=on
  Discrete Constant2 : dspsrcs4/DSP Constant  SystemSampleTime=-1  Value=pi2  SampleMode=Discrete  discreteOutput=Sample-based (interpret vectors as 1-D)  continuousOutput=Sample-based  sampTime=1/8000  framePeriod=1/8000  dataType=Inherit via back propagation  isSigned=on  wordLen=16  udDataType=sfix(16)  fracBitsMode=Best precision  numFracBits=15  InterpretAs1D=on  Ts=1/8000  FramebasedOutput=off
      settings: SourceProductName=DSP System Toolbox  SourceProductBaseCode=DS  additionalParams=on
  Math Function : Math  Operator=mod  SaturateOnIntegerOverflow=on
  Sensitivity : Gain  Gain=Kc*pi2*ts  SaturateOnIntegerOverflow=on  OutDataTypeStr=Inherit: Same as input  ParamDataTypeStr=Inherit: Same as input
  Sensitivity2 : Gain  Gain=Ac  SaturateOnIntegerOverflow=on  OutDataTypeStr=Inherit: Same as input  ParamDataTypeStr=Inherit: Same as input
  Sum1 : Sum  Inputs=+++  SaturateOnIntegerOverflow=on  InputSameDT=on  OutDataTypeStr=Inherit: Same as first input
  Trigonometric Function : Trigonometry  Operator=cos
  Unit Delay : UnitDelay  InitialCondition=Ph  SampleTime=ts
  out_1 : Outport  InitialOutput=0
  wires:
  Discrete Constant1/1 -> Sum1/2
  Sensitivity2/1 -> out_1/1
  Trigonometric Function/1 -> Sensitivity2/1
  Unit Delay/1 -> Trigonometric Function/1, Sum1/3
  Sensitivity/1 -> Sum1/1
  in_1/1 -> Sensitivity/1
  Math Function/1 -> Unit Delay/1
  Sum1/1 -> Math Function/1
  Discrete Constant2/1 -> Math Function/2
